simulink library "calcUCB"  (R2018b)
settings: Solver=VariableStepAuto  StartTime=0.0  StopTime=10.0  RelTol=1e-3
undefined symbols (not defined in the file or in its folder): postVarGain, predMeanGain
settings Model: Creator=Ayaz  LastModifiedBy=Ayaz
settings DataIOCC: ReturnWorkspaceOutputs=on

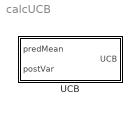
== system calcUCB ==
  UCB : Subsystem  mask{predMeanGain=predMeanGain, postVarGain=postVarGain}
      mask prompts: predMeanGain "Prediction mean gain"; postVarGain "Posterior variance gain"
      mask TypeOptions predMeanGain: Gain/Gain
      mask TypeOptions postVarGain: Gain1/Gain

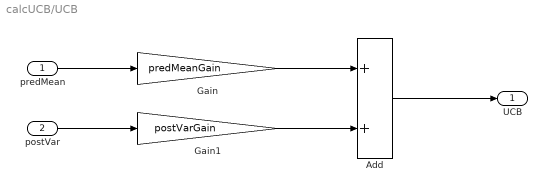
== system calcUCB/UCB ==
  predMean : Inport
  postVar : Inport  Port=2
  Add : Sum
  Gain : Gain  Gain=predMeanGain
  Gain1 : Gain  Gain=postVarGain
  UCB : Outport
  wires:
  predMean/1 -> Gain/1
  postVar/1 -> Gain1/1
  Gain/1 -> Add/1
  Gain1/1 -> Add/2
  Add/1 -> UCB/1
